simulink library "attitude_estimation_lib"  (R2018b)
settings: Solver=VariableStepAuto  StartTime=0.0  StopTime=10.0  RelTol=1e-3
undefined symbols (not defined in the file or in its folder): fswParams
libraries: extended_kalman_filter_lib x1, triad_coarse_estimator x1
settings Model: Creator=sexymathemagician  LastModifiedBy=devantormey
settings SFSimCC: SimUseLocalCustomCode=off
settings RTWCC: RTWUseLocalCustomCode=off
settings CodeAppCC: StateflowObjectComments=on

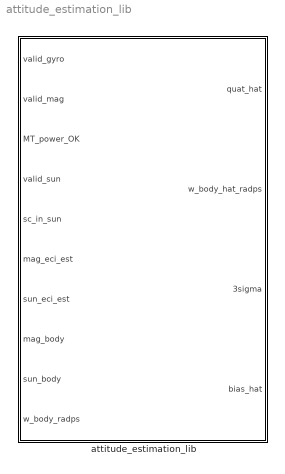
== system attitude_estimation_lib ==
  attitude_estimation_lib : Subsystem

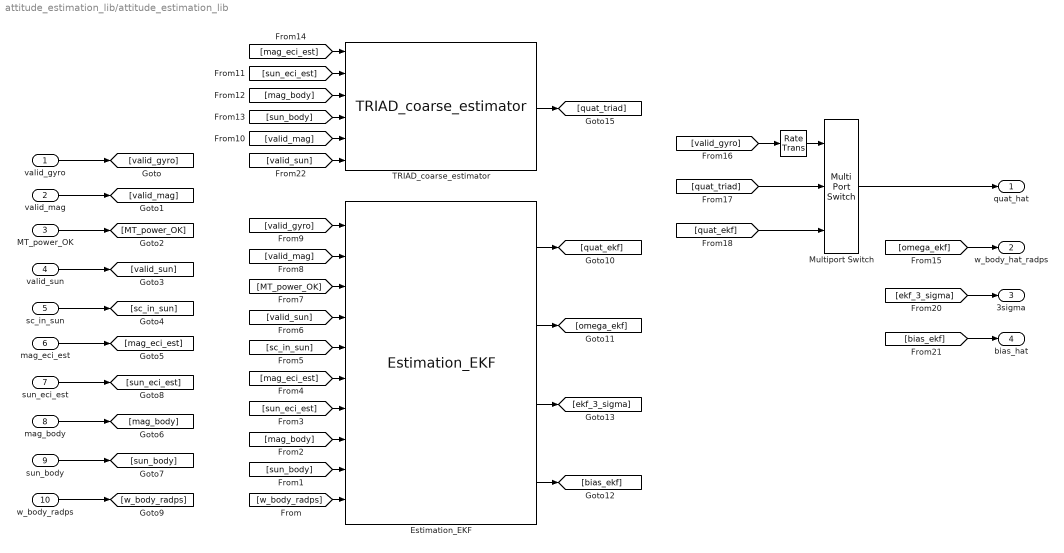
== system attitude_estimation_lib/attitude_estimation_lib ==
  valid_gyro : Inport
  valid_mag : Inport  Port=2
  MT_power_OK : Inport  Port=3
  "valid_sun " : Inport  Port=4
  sc_in_sun : Inport  Port=5
  mag_eci_est : Inport  Port=6
  sun_eci_est : Inport  Port=7
  mag_body : Inport  Port=8
  sun_body : Inport  Port=9
  w_body_radps : Inport  Port=10
  " " : RateTransition  InitialCondition=fswParams.estimation.ic.rt_valid_gyro  OutPortSampleTime=fswParams.estimation.sample_time_s
  "Estimation_EKF " : extended_kalman_filter_lib/Estimation_EKF   SystemSampleTime=-1
      link override " ": InitialCondition=fswParams.estimation.ic.rt_valid_gyro
  Multiport Switch : MultiPortSwitch  DataPortOrder=Zero-based contiguous  Inputs=2  zeroidx=on
  TRIAD_coarse_estimator : triad_coarse_estimator/TRIAD_coarse_estimator  SystemSampleTime=-1
  quat_hat : Outport
  w_body_hat_radps : Outport  Port=2
  3sigma : Outport  Port=3
  bias_hat : Outport  Port=4
  wires:
  valid_gyro/1 -> [valid_gyro]
  valid_mag/1 -> [valid_mag]
  "valid_sun "/1 -> [valid_sun]
  mag_body/1 -> [mag_body]
  sun_body/1 -> [sun_body]
  MT_power_OK/1 -> [MT_power_OK]
  [bias_ekf] -> bias_hat/1
  [ekf_3_sigma] -> 3sigma/1
  [omega_ekf] -> w_body_hat_radps/1
  sc_in_sun/1 -> [sc_in_sun]
  mag_eci_est/1 -> [mag_eci_est]
  sun_eci_est/1 -> [sun_eci_est]
  [valid_gyro] -> "Estimation_EKF "/1
  [valid_mag] -> "Estimation_EKF "/2
  [MT_power_OK] -> "Estimation_EKF "/3
  [valid_sun] -> "Estimation_EKF "/4
  [sc_in_sun] -> "Estimation_EKF "/5
  [mag_eci_est] -> "Estimation_EKF "/6
  [sun_eci_est] -> "Estimation_EKF "/7
  [mag_body] -> "Estimation_EKF "/8
  [sun_body] -> "Estimation_EKF "/9
  w_body_radps/1 -> [w_body_radps]
  [w_body_radps] -> "Estimation_EKF "/10
  [mag_eci_est] -> TRIAD_coarse_estimator/1
  [sun_eci_est] -> TRIAD_coarse_estimator/2
  [mag_body] -> TRIAD_coarse_estimator/3
  [sun_body] -> TRIAD_coarse_estimator/4
  [valid_mag] -> TRIAD_coarse_estimator/5
  [valid_sun] -> TRIAD_coarse_estimator/6
  TRIAD_coarse_estimator/1 -> [quat_triad]
  "Estimation_EKF "/1 -> [quat_ekf]
  [valid_gyro] -> " "/1
  "Estimation_EKF "/4 -> [bias_ekf]
  "Estimation_EKF "/3 -> [ekf_3_sigma]
  "Estimation_EKF "/2 -> [omega_ekf]
  " "/1 -> Multiport Switch/1
  [quat_triad] -> Multiport Switch/2
  [quat_ekf] -> Multiport Switch/3
  Multiport Switch/1 -> quat_hat/1
